simulink model "Vehicle_definitivo_validazione_2"  (R2025b)
settings: Solver=ode4  StartTime=0.0  StopTime=30  FixedStep=0.001  RelTol=1e-3
undefined symbols (not defined in the file): car, new_lotus_bump, new_lotus_roll, new_lotus_steer, posRef, rad, s, Tau_1, Tau_2, Tau_3, Tau_4, yawRef
libraries: aerolibconvert2 x28, simulink_extras x16, simulink x12, slpidlib x2, mpclib x1
(part 3 of 13)

== system Vehicle_definitivo_validazione_2/Con relaxation/Vehicle/Powertrain/Electric Motor ==
  tps_EM : Inport
  omega wheels : Inport  Port=2
  2-D Lookup Table : Lookup_n-D  BreakpointsForDimension1=[0;5415.9399999999996;5455.8699999999999;5494.6300000000001;5524.8000000000002;5801.2200000000003;6194.8599999999997;6620.2799999999997;6996.5;7478.6599999999999;8072.5500000000002;8891.9799999999996;8998.9200000000001;9966.8600000000006;10994.200000000001;11872.6;13016.16;13972.65;15994.85]  BreakpointsForDimension2=[0;0.25;0.29999999999999999;0.34999999999999998;0.40000000000000002;0.45000000000000001;0.5;0.59999999999999998;0.69999999999999996;0.80000000000000004;1]  Table=[0 1.72854705 2.07425646 2.41996587 2.7656752899999999 3.1113846999999999 3.4570941099999999 4.1485129299999999 4.8399317000000002 5.5313505699999999 6.9141880000000002;0 1.72755429 2.0730651500000001 2.4185760100000002 2.7640868599999999 3.10959772 3.4551085800000001 4.1461303000000003 4.8371519999999997 5.5281737299999998 6.9102170000000003;0 1.7172173399999999 2.0606608099999999 2.4041042799999999 2.7475477499999998 3.0909912099999999 3.4344346799999999 4.1213216199999998 4.8082086000000004 5.4950954899999997 6.8688690000000001;0 1.7114327 2.0537192399999999 2.3960057799999999 2.7382923199999998 3.0805788600000001 3.4228654000000001 4.1074384799999999 4.7920116000000004 5.4765846399999996 6.8457309999999998;0 1.7057860899999999 2.0469433100000001 2.3881005200000001 2.72925774 3.0704149599999999 3.4115721799999998 4.0938866100000002 4.7762010000000004 5.45851548 6.8231440000000001;0 1.65353861 1.9842463299999999 2.3149540499999999 2.6456617699999998 2.9763694900000002 3.3070772100000001 3.96849265 4.6299080999999997 5.2913235399999996 6.6141540000000001;0 1.57836584 1.89403901 2.2097121799999999 2.5253853500000001 2.8410585199999998 3.15673168 3.7880780199999999 4.4194243999999996 5.0507707000000002 6.3134629999999996;0 1.5001957400000001 1.80023489 2.10027404 2.4003131899999999 2.7003523399999998 3.0003914800000002 3.6004697800000001 4.2005480999999998 4.8006263699999998 6.0007830000000002;0 1.43080228 1.71696274 2.0031231900000002 2.2892836499999998 2.5754440999999999 2.86160456 3.4339254700000001 4.0062464000000002 4.5785672899999996 5.7232089999999998;0 1.34976662 1.6197199499999999 1.8896732700000001 2.1596266000000002 2.4295799200000001 2.69953325 3.2394398899999999 3.7793464999999999 4.3192531900000004 5.3990660000000004;0 1.24874098 1.49848917 1.74823737 1.99798556 2.24773376 2.4974819500000001 2.9969783400000001 3.4964746999999998 3.9959711200000001 4.9949640000000004;0 1.1245459799999999 1.3494551800000001 1.57436438 1.79927357 2.0241827699999999 2.2490919699999998 2.6989103600000002 3.1487288000000002 3.5985471499999999 4.4981840000000002;0 1.11256427 1.3350771299999999 1.5575899799999999 1.7801028299999999 2.0026156899999998 2.22512854 2.67015425 3.1151800000000001 3.5602056700000002 4.4502569999999997;0 0.98525799000000003 1.18230959 1.3793611800000001 1.5764127800000001 1.7734643800000001 1.9705159800000001 2.3646191700000001 2.7587223999999999 3.1528255600000001 3.9410319999999999;0 0.88127745999999996 1.0575329600000001 1.23378845 1.41004394 1.5862994399999999 1.7625549300000001 2.1150659100000002 2.4675769000000001 2.8200878899999999 3.5251100000000002;0 0.79965012999999996 0.95958014999999997 1.11951018 1.2794402 1.43937023 1.59930025 1.9191602999999999 2.2390203999999998 2.5588804000000001 3.198601;0 0.70417978000000003 0.84501572999999996 0.98585168999999995 1.1266876400000001 1.2675236000000001 1.4083595600000001 1.6900314700000001 1.9717034 2.2533752900000001 2.816719;0 0.63972525999999996 0.76767032000000002 0.89561537000000002 1.0235604199999999 1.15150547 1.2794505300000001 1.5353406300000001 1.7912307000000001 2.0471208399999998 2.5589010000000001;0 0.51010575999999996 0.61212690999999997 0.71414805999999997 0.81616922000000003 0.91819037000000003 1.0202115199999999 1.2242538199999999 1.4282961000000001 1.6323384299999999 2.0404230000000001]  InternalRulePriority=Speed  RndMeth=Simplest
      settings: InputPortMap=u0,u1
  2-D Lookup Table1 : Lookup_n-D  BreakpointsForDimension1=[0;5415.9399999999996;5455.8699999999999;5494.6300000000001;5524.8000000000002;5801.2200000000003;6194.8599999999997;6620.2799999999997;6996.5;7478.6599999999999;8072.5500000000002;8891.9799999999996;8998.9200000000001;9966.8600000000006;10994.200000000001;11872.6;13016.16;13972.65;15994.85]  BreakpointsForDimension2=[0;0.25;0.29999999999999999;0.34999999999999998;0.40000000000000002;0.45000000000000001;0.5;0.59999999999999998;0.69999999999999996;0.80000000000000004;1]  Table=[0 1.72854705 2.07425646 2.41996587 2.7656752899999999 3.1113846999999999 3.4570941099999999 4.1485129299999999 4.8399317000000002 5.5313505699999999 6.9141880000000002;0 1.72755429 2.0730651500000001 2.4185760100000002 2.7640868599999999 3.10959772 3.4551085800000001 4.1461303000000003 4.8371519999999997 5.5281737299999998 6.9102170000000003;0 1.7172173399999999 2.0606608099999999 2.4041042799999999 2.7475477499999998 3.0909912099999999 3.4344346799999999 4.1213216199999998 4.8082086000000004 5.4950954899999997 6.8688690000000001;0 1.7114327 2.0537192399999999 2.3960057799999999 2.7382923199999998 3.0805788600000001 3.4228654000000001 4.1074384799999999 4.7920116000000004 5.4765846399999996 6.8457309999999998;0 1.7057860899999999 2.0469433100000001 2.3881005200000001 2.72925774 3.0704149599999999 3.4115721799999998 4.0938866100000002 4.7762010000000004 5.45851548 6.8231440000000001;0 1.65353861 1.9842463299999999 2.3149540499999999 2.6456617699999998 2.9763694900000002 3.3070772100000001 3.96849265 4.6299080999999997 5.2913235399999996 6.6141540000000001;0 1.57836584 1.89403901 2.2097121799999999 2.5253853500000001 2.8410585199999998 3.15673168 3.7880780199999999 4.4194243999999996 5.0507707000000002 6.3134629999999996;0 1.5001957400000001 1.80023489 2.10027404 2.4003131899999999 2.7003523399999998 3.0003914800000002 3.6004697800000001 4.2005480999999998 4.8006263699999998 6.0007830000000002;0 1.43080228 1.71696274 2.0031231900000002 2.2892836499999998 2.5754440999999999 2.86160456 3.4339254700000001 4.0062464000000002 4.5785672899999996 5.7232089999999998;0 1.34976662 1.6197199499999999 1.8896732700000001 2.1596266000000002 2.4295799200000001 2.69953325 3.2394398899999999 3.7793464999999999 4.3192531900000004 5.3990660000000004;0 1.24874098 1.49848917 1.74823737 1.99798556 2.24773376 2.4974819500000001 2.9969783400000001 3.4964746999999998 3.9959711200000001 4.9949640000000004;0 1.1245459799999999 1.3494551800000001 1.57436438 1.79927357 2.0241827699999999 2.2490919699999998 2.6989103600000002 3.1487288000000002 3.5985471499999999 4.4981840000000002;0 1.11256427 1.3350771299999999 1.5575899799999999 1.7801028299999999 2.0026156899999998 2.22512854 2.67015425 3.1151800000000001 3.5602056700000002 4.4502569999999997;0 0.98525799000000003 1.18230959 1.3793611800000001 1.5764127800000001 1.7734643800000001 1.9705159800000001 2.3646191700000001 2.7587223999999999 3.1528255600000001 3.9410319999999999;0 0.88127745999999996 1.0575329600000001 1.23378845 1.41004394 1.5862994399999999 1.7625549300000001 2.1150659100000002 2.4675769000000001 2.8200878899999999 3.5251100000000002;0 0.79965012999999996 0.95958014999999997 1.11951018 1.2794402 1.43937023 1.59930025 1.9191602999999999 2.2390203999999998 2.5588804000000001 3.198601;0 0.70417978000000003 0.84501572999999996 0.98585168999999995 1.1266876400000001 1.2675236000000001 1.4083595600000001 1.6900314700000001 1.9717034 2.2533752900000001 2.816719;0 0.63972525999999996 0.76767032000000002 0.89561537000000002 1.0235604199999999 1.15150547 1.2794505300000001 1.5353406300000001 1.7912307000000001 2.0471208399999998 2.5589010000000001;0 0.51010575999999996 0.61212690999999997 0.71414805999999997 0.81616922000000003 0.91819037000000003 1.0202115199999999 1.2242538199999999 1.4282961000000001 1.6323384299999999 2.0404230000000001]  InternalRulePriority=Speed  RndMeth=Simplest
      settings: InputPortMap=u0,u1
  Angular Velocity Conversion : aerolibconvert2/Angular Velocity Conversion  IU=rpm  OU=rad/s
  Angular Velocity Conversion1 : aerolibconvert2/Angular Velocity Conversion  IU=rad/s  OU=rpm
  Angular Velocity Conversion2 : aerolibconvert2/Angular Velocity Conversion  IU=rpm  OU=rad/s
  Demux : Demux
  Gain : Gain  Gain=car.Tau_EM
  Gain1 : Gain  Gain=car.Tau_EM
  Gain3 : Gain  Gain=car.Tau_EM
  Integrator : Integrator  InitialCondition=1  LimitOutput=on  UpperSaturationLimit=1  LowerSaturationLimit=0
  Limiter1 : Saturate  UpperLimit=16000  LowerLimit=0
  MATLAB Function : MATLAB Function  TreatAsAtomicUnit=on
  T_FR : Outport
  T_FL : Outport  Port=2
  wires:
  2-D Lookup Table/1 -> Gain/1, MATLAB Function/1(T_FR)
  2-D Lookup Table1/1 -> MATLAB Function/2(T_FL), Gain1/1
  omega wheels/1 -> Angular Velocity Conversion1/1
  Angular Velocity Conversion1/1 -> Gain3/1
  Gain3/1 -> Limiter1/1
  Gain/1 -> T_FR/1
  Gain1/1 -> T_FL/1
  tps_EM/1 -> 2-D Lookup Table1/2, 2-D Lookup Table/2
  Limiter1/1 -> Demux/1
  Demux/1 -> 2-D Lookup Table/1, Angular Velocity Conversion/1
  Demux/2 -> Angular Velocity Conversion2/1, 2-D Lookup Table1/1
  MATLAB Function/1(SoC_dot) -> Integrator/1
  Integrator/1 -> MATLAB Function/5(SoC)
  Angular Velocity Conversion/1 -> MATLAB Function/3(w_FR)
  Angular Velocity Conversion2/1 -> MATLAB Function/4(w_FL)

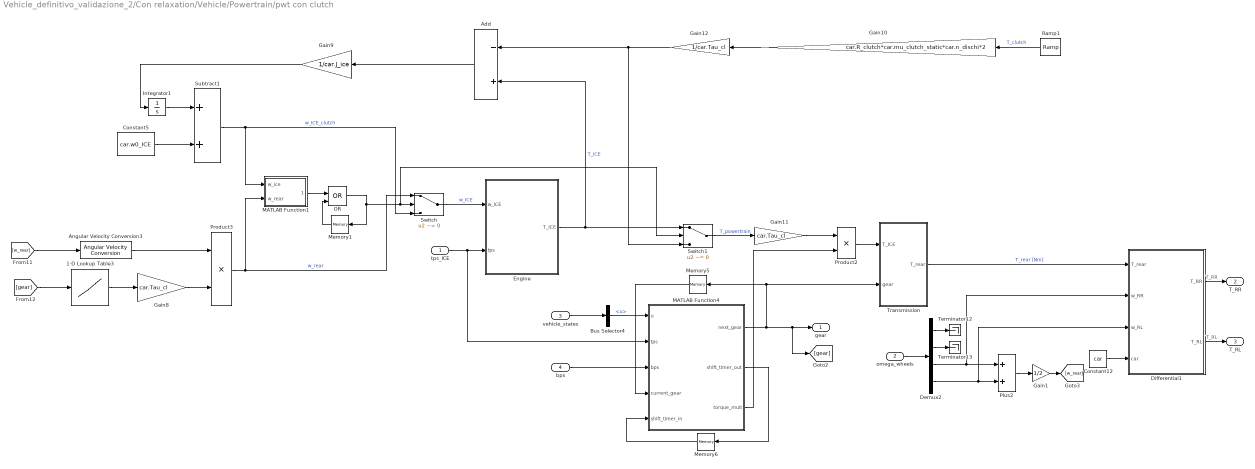
== system Vehicle_definitivo_validazione_2/Con relaxation/Vehicle/Powertrain/pwt con clutch ==
  tps_ICE : Inport
  omega_wheels : Inport  Port=2
  vehicle_states : Inport  Port=3
  bps : Inport  Port=4
  1-D Lookup Table3 : Lookup_n-D  NumberOfTableDimensions=1  BreakpointsForDimension1=[1;2;3;4]  Table=[Tau_1; Tau_2; Tau_3; Tau_4]  InternalRulePriority=Speed  RndMeth=Simplest
  Add : Sum  Inputs=-+
  Angular Velocity Conversion3 : aerolibconvert2/Angular Velocity Conversion  IU=rad/s  OU=rpm
  Bus Selector4 : BusSelector  OutputSignals=velocities.u
  Constant12 : Constant  Value=car  OutDataTypeStr=Bus: slBus1
  Constant5 : Constant  Value=car.w0_ICE
  Demux2 : Demux
  Differential1 : MATLAB Function  TreatAsAtomicUnit=on
  Engine : Subsystem
  Gain1 : Gain  Gain=1/2
  Gain10 : Gain  Gain=car.R_clutch*car.mu_clutch_static*car.n_dischi*2
  Gain11 : Gain  Gain=car.Tau_cl
  Gain12 : Gain  Gain=1/car.Tau_cl
  Gain8 : Gain  Gain=car.Tau_cl
  Gain9 : Gain  Gain=1/car.J_ice
  Integrator1 : Integrator
  MATLAB Function1 : MATLAB Function  TreatAsAtomicUnit=on
  MATLAB Function4 : MATLAB Function  TreatAsAtomicUnit=on
  Memory1 : Memory
  Memory5 : Memory  InitialCondition=2
  Memory6 : Memory
  OR : Logic  Operator=OR  IconShape=distinctive  AllPortsSameDT=off  OutDataTypeStr=boolean
  Plus2 : Sum
  Product2 : Product
  Product3 : Product
  Ramp1 : simulink/Sources/Ramp  slope=5000  start=0  InitialOutput=671
  Subtract1 : Sum
  Switch : Switch  Criteria=u2 ~= 0  Threshold=50  SaturateOnIntegerOverflow=off  InputSameDT=off
  Switch1 : Switch  Criteria=u2 ~= 0  Threshold=50  SaturateOnIntegerOverflow=off  InputSameDT=off
  Terminator12 : Terminator
  Terminator13 : Terminator
  Transmission : Subsystem
  gear : Outport
  T_RR : Outport  Port=2
  T_RL : Outport  Port=3
  wires:
  Ramp1/1 -> Gain10/1  "T_clutch"
  MATLAB Function1/1(condizione) -> OR/1
  [gear] -> 1-D Lookup Table3/1
  Gain10/1 -> Gain12/1
  Angular Velocity Conversion3/1 -> Product3/1
  [w_rear] -> Angular Velocity Conversion3/1
  Gain12/1 -> Switch1/3, Add/1
  Integrator1/1 -> Subtract1/1
  Switch/1 -> Engine/1(w_ICE)  "w_ICE"
  Subtract1/1 -> Switch/3, MATLAB Function1/1(w_ice)  "w_ICE_clutch"
  Switch1/1 -> Gain11/1  "T_powertrain"
  Constant5/1 -> Subtract1/2
  Memory1/1 -> OR/2
  tps_ICE/1 -> Engine/2(tps), MATLAB Function4/2(tps)
  Add/1 -> Gain9/1
  Memory5/1 -> MATLAB Function4/4(current_gear)
  bps/1 -> MATLAB Function4/3(bps)
  OR/1 -> Memory1/1, Switch/2, Switch1/2
  vehicle_states/1 -> Bus Selector4/1
  Demux2/1 -> Terminator12/1
  Gain8/1 -> Product3/2
  Gain1/1 -> [w_rear]
  1-D Lookup Table3/1 -> Gain8/1
  Plus2/1 -> Gain1/1
  omega_wheels/1 -> Demux2/1
  MATLAB Function4/2(shift_timer_out) -> Memory6/1
  Transmission/1(T_rear) -> Differential1/1(T_rear)  "T_rear [Nm]"
  Memory6/1 -> MATLAB Function4/5(shift_timer_in)
  Demux2/2 -> Terminator13/1
  Demux2/4 -> Differential1/3(w_RL), Plus2/2
  Bus Selector4/1 -> MATLAB Function4/1(u)  "<u>"
  Demux2/3 -> Differential1/2(w_RR), Plus2/1
  MATLAB Function4/1(next_gear) -> Memory5/1, Transmission/2(gear), gear/1, [gear]
  Product3/1 -> MATLAB Function1/2(w_rear), Switch/1  "w_rear"
  Gain11/1 -> Product2/1
  MATLAB Function4/3(torque_mult) -> Product2/2
  Engine/1(T_ICE) -> Add/2, Switch1/1  "T_ICE"
  Gain9/1 -> Integrator1/1
  Product2/1 -> Transmission/1(T_ICE)
  Differential1/1(T_RR) -> T_RR/1  "T_RR"
  Constant12/1 -> Differential1/4(car)
  Differential1/2(T_RL) -> T_RL/1  "T_RL"

== system Vehicle_definitivo_validazione_2/Con relaxation/Vehicle/Powertrain/pwt senza clutch ==
  tps_ICE : Inport
  vehicle_states : Inport  Port=2
  bps : Inport  Port=3
  omega_wheels : Inport  Port=4
  1-D Lookup Table1 : Lookup_n-D  NumberOfTableDimensions=1  BreakpointsForDimension1=[1;2;3;4]  Table=[Tau_1; Tau_2; Tau_3; Tau_4]  InternalRulePriority=Speed  RndMeth=Simplest
  Angular Velocity Conversion1 : aerolibconvert2/Angular Velocity Conversion  IU=rad/s  OU=rpm
  Bus Selector3 : BusSelector  OutputSignals=Veh_States.velocities.u
  Constant12 : Constant  Value=car  OutDataTypeStr=Bus: slBus1
  Demux : Demux
  Differential : MATLAB Function  TreatAsAtomicUnit=on
  Engine : Subsystem
  Gain1 : Gain  Gain=1/2
  Gain2 : Gain  Gain=car.Tau_cl
  Gain5 : Gain  Gain=car.Tau_cl
  Gearbox : MATLAB Function  TreatAsAtomicUnit=on
  Memory : Memory  InitialCondition=2
  Memory3 : Memory
  Plus : Sum
  Product : Product
  Product1 : Product
  Terminator : Terminator
  Terminator1 : Terminator
  Transmission : Subsystem
  T_RR : Outport
  T_RL : Outport  Port=2
  gear : Outport  Port=3
  wires:
  Memory/1 -> Gearbox/4(current_gear)
  Gain5/1 -> Product1/2
  vehicle_states/1 -> Bus Selector3/1
  Angular Velocity Conversion1/1 -> Product1/1
  Gearbox/3(shift_timer_out) -> Memory3/1
  Memory3/1 -> Gearbox/5(shift_timer_in)
  bps/1 -> Gearbox/3(bps)  "bps"
  1-D Lookup Table1/1 -> Gain5/1
  Bus Selector3/1 -> Gearbox/1(u)  "<u>"
  Gearbox/1(next_gear) -> Memory/1, Transmission/2(gear), gear/1, [gear]  "gear"
  [gear] -> 1-D Lookup Table1/1
  Transmission/1(T_rear) -> Differential/1(T_rear)  "T_rear [Nm]"
  tps_ICE/1 -> Gearbox/2(tps), Engine/2(tps)  "tps"
  Product/1 -> Transmission/1(T_ICE)
  Engine/1(T_ICE) -> Gain2/1  "T_ICE"
  Product1/1 -> Engine/1(w_ICE)  "w_ICE"
  Gearbox/2(torque_mult) -> Product/2
  Gain2/1 -> Product/1
  Plus/1 -> Gain1/1
  Demux/3 -> Plus/1, [w_RR]
  Gain1/1 -> Angular Velocity Conversion1/1
  Demux/4 -> [w_RL], Plus/2
  omega_wheels/1 -> Demux/1
  Demux/1 -> Terminator/1  "w_front"
  Demux/2 -> Terminator1/1
  Differential/1(T_RR) -> T_RR/1  "T_RR"
  Differential/2(T_RL) -> T_RL/1  "T_RL"
  [w_RR] -> Differential/2(w_RR)
  [w_RL] -> Differential/3(w_RL)
  Constant12/1 -> Differential/4(car)

== system Vehicle_definitivo_validazione_2/Driver in the Loop/Vehicle/Brakes/Front Caliper ==
  P_Front : Inport
  Gain : Gain  Gain=4
  Pad Friction : Gain  Gain=car.brakepad_friction_coeff
  Piston area : Gain  Gain=car.area_front_piston
  brake radius : Gain  Gain=car.brake_radius_front
  from bar to Pascal : Gain  Gain=100000
  T_brake_FR : Outport
  T_brake_FL : Outport  Port=2
  wires:
  P_Front/1 -> from bar to Pascal/1
  Pad Friction/1 -> brake radius/1
  brake radius/1 -> T_brake_FR/1, T_brake_FL/1
  from bar to Pascal/1 -> Gain/1
  Piston area/1 -> Pad Friction/1
  Gain/1 -> Piston area/1

== system Vehicle_definitivo_validazione_2/Driver in the Loop/Vehicle/Brakes/Proportional Valve ==
  P_rear : Inport
  2-D Lookup Table : Lookup_n-D  BreakpointsForDimension1=[0;3.4473799999999999;6.8947599999999998;10.342140000000001;13.78952;17.236899999999999;20.684280000000001;24.13166;27.579039999999999;31.026420000000002;34.473799999999997;37.92118;41.368560000000002;44.815939999999998;48.26332;51.710700000000003;55.158079999999998;58.605460000000001;62.052840000000003;65.500219999999999;68.947599999999994;72.394980000000004;75.842359999999999;79.289739999999995;82.737120000000004]  BreakpointsForDimension2=[1;2;3;4;5;6;7]  Table=[0 0 0 0 0 0 0;3.4473799999999999 3.4473799999999999 3.4473799999999999 3.4473799999999999 3.4473799999999999 3.4473799999999999 3.4473799999999999;6.8947599999999998 6.8947599999999998 6.8947599999999998 6.8947599999999998 6.8947599999999998 6.8947599999999998 6.8947599999999998;10.342140000000001 10.342140000000001 10.342140000000001 10.342140000000001 10.342140000000001 10.342140000000001 10.342140000000001;11.49126667 13.78952 13.78952 13.78952 13.78952 13.78952 13.78952;12.64039333 17.236899999999999 17.236899999999999 17.236899999999999 17.236899999999999 17.236899999999999 17.236899999999999;13.78952 20.684280000000001 20.684280000000001 20.684280000000001 20.684280000000001 20.684280000000001 20.684280000000001;14.938646670000001 21.833406669999999 24.13166 24.13166 24.13166 24.13166 24.13166;16.087773330000001 22.982533329999999 27.579039999999999 27.579039999999999 27.579039999999999 27.579039999999999 27.579039999999999;17.236899999999999 24.13166 31.026420000000002 31.026420000000002 31.026420000000002 31.026420000000002 31.026420000000002;18.38602667 25.280786670000001 34.473799999999997 34.473799999999997 34.473799999999997 34.473799999999997 34.473799999999997;19.53515333 26.429913330000002 35.458765710000002 37.92118 37.92118 37.92118 37.92118;20.684280000000001 27.579039999999999 36.44373143 41.368560000000002 41.368560000000002 41.368560000000002 41.368560000000002;21.833406669999999 28.72816667 37.428697139999997 42.517686670000003 44.815939999999998 44.815939999999998 44.815939999999998;22.982533329999999 29.877293330000001 38.413662860000002 43.666813329999997 48.26332 48.26332 48.26332;24.13166 31.026420000000002 39.39862857 44.815939999999998 51.710700000000003 51.710700000000003 51.710700000000003;25.280786670000001 32.175546670000003 40.383594289999998 45.965066669999999 52.859826669999997 55.158079999999998 55.158079999999998;26.429913330000002 33.324673330000003 41.368560000000002 47.114193329999999 54.008953329999997 58.605460000000001 58.605460000000001;27.579039999999999 34.473799999999997 42.35352571 48.26332 55.158079999999998 62.052840000000003 62.052840000000003;28.72816667 35.622926669999998 43.338491429999998 49.412446670000001 56.307206669999999 63.201966669999997 65.500219999999999;29.877293330000001 36.772053329999999 44.323457140000002 50.561573330000002 57.45633333 64.351093329999998 68.947599999999994;31.026420000000002 37.92118 45.30842286 51.710700000000003 58.605460000000001 65.500219999999999 70.671289999999999;32.175546670000003 39.070306670000001 46.293388569999998 52.859826669999997 59.754586670000002 66.64934667 72.394980000000004;33.324673330000003 40.219433330000001 47.278354290000003 54.008953329999997 60.903713330000002 67.798473329999993 74.118669999999995;34.473799999999997 41.368560000000002 48.26332 55.158079999999998 62.052840000000003 68.947599999999994 75.842359999999999]  InternalRulePriority=Speed  RndMeth=Simplest
      settings: InputPortMap=u0,u1
  Constant : Constant  Value=car.prop_valve_pos
  p_rear_mod : Outport
  wires:
  P_rear/1 -> 2-D Lookup Table/1
  Constant/1 -> 2-D Lookup Table/2
  2-D Lookup Table/1 -> p_rear_mod/1

== system Vehicle_definitivo_validazione_2/Driver in the Loop/Vehicle/Brakes/Rear Caliper ==
  P_rear : Inport
  Gain : Gain  Gain=2
  Pad Friction : Gain  Gain=car.brakepad_friction_coeff
  Piston area : Gain  Gain=car.area_rear_piston
  brake radius_rear : Gain  Gain=car.brake_radius_rear
  from bar to Pascal : Gain  Gain=100000
  T_brake_RR : Outport
  T_brake_RL : Outport  Port=2
  wires:
  P_rear/1 -> from bar to Pascal/1
  Pad Friction/1 -> brake radius_rear/1
  brake radius_rear/1 -> T_brake_RL/1, T_brake_RR/1
  from bar to Pascal/1 -> Gain/1
  Gain/1 -> Piston area/1
  Piston area/1 -> Pad Friction/1

== system Vehicle_definitivo_validazione_2/Driver in the Loop/Vehicle/Chassis/Aeromaps ==
  Ride_height : Inport
  Constant : Constant  Value=car.Cx
  Constant1 : Constant  Value=car.Cz
  Constant2 : Constant  Value=car.x_cp
  Demux : Demux
  Mux : Mux  Inputs=3
  aero_coeff : Outport
  wires:
  Constant/1 -> Mux/1
  Constant1/1 -> Mux/2
  Ride_height/1 -> Demux/1
  Mux/1 -> aero_coeff/1
  Constant2/1 -> Mux/3

== system Vehicle_definitivo_validazione_2/Driver in the Loop/Vehicle/Chassis/Damper ==
  susp_vel_ground : Inport
  IR : Inport  Port=2
  Demux : Demux
  FL : Subsystem
  FR : Subsystem
  Mux : Mux
  Product : Product
  Product1 : Product
  RL : Subsystem
  RR : Subsystem
  F_damper : Outport
  wires:
  IR/1 -> Product1/2, Product/2
  Product/1 -> Demux/1
  Demux/1 -> FR/1(V_FR)
  FR/1(F_FR) -> Mux/1  "F_FR"
  Mux/1 -> Product1/1
  Demux/2 -> FL/1(V_FL)
  FL/1(F_FL) -> Mux/2  "F_FL"
  Demux/3 -> RR/1(V_RR)
  RR/1(F_RR) -> Mux/3  "F_RR"
  Demux/4 -> RL/1(V_RL)
  RL/1(F_RL) -> Mux/4  "F_RL"
  susp_vel_ground/1 -> Product/1
  Product1/1 -> F_damper/1

== system Vehicle_definitivo_validazione_2/Driver in the Loop/Vehicle/Chassis/kinematics ==
  Steer_Angle : Inport
  Wheel_Travel : Inport  Port=2
  Add{,1..5} (6 alike) : Sum
  Constant : Constant  Value=car.lf
  Constant1 : Constant  Value=car.lr
  Constant2 : Constant  Value=car.h_cog
  Constant3 : Constant  Value=0.03
  Constant4 : Constant  Value=0.04
  Degrees to Radians : simulink_extras/Transformations/Degrees to Radians
  Demux : Demux
  FL : Subsystem
  FR : Subsystem
  Gain{,1..3} (4 alike) : Gain  Gain=0.5
  Gain4 : Gain  Gain=-1
  Mux : Mux  Inputs=11
  Mux1 : Mux
  Mux2 : Mux
  Mux3 : Mux
  RL : Subsystem
  RR : Subsystem
  Subsystem : Subsystem
  Subsystem1 : Subsystem
  Subtract : Sum  Inputs=-+
  Subtract1 : Sum  Inputs=-+
  kin_dyn : Outport
  anti% : Outport  Port=2
  camber : Outport  Port=3
  toe : Outport  Port=4
  wires:
  Demux/1 -> FR/1(Wheel_Travel), Subtract/1, Add/1
  Add/1 -> Gain/1
  Gain/1 -> Subsystem/1(Heave_F)
  Subtract/1 -> Subsystem/2(Roll_F)
  Demux/3 -> Subtract1/1, Add1/1, RR/1(Wheel_Travel)
  Demux/4 -> RL/1(Wheel_Travel), Add1/2, Subtract1/2
  Add1/1 -> Gain1/1
  Steer_Angle/1 -> FR/2(Steer_Angle), Gain4/1
  Demux/2 -> FL/2(Wheel_Travel), Add/2, Subtract/2
  Mux/1 -> kin_dyn/1
  FR/3(IR_FR) -> Mux/1
  FL/3(IR_FL) -> Mux/2
  RR/3(IR_RR) -> Mux/3
  RL/3(IR_RL) -> Mux/4
  Subsystem/2(tf) -> Mux/5
  Subsystem1/2(tr) -> Mux/6
  FR/1(wb_FR) -> Add2/1
  FL/1(wb_FL) -> Add2/2
  Add2/1 -> Gain2/1
  Gain2/1 -> Add3/1
  Constant/1 -> Add3/2
  Add3/1 -> Mux/7
  Constant1/1 -> Add5/2
  Gain3/1 -> Add5/1
  Add4/1 -> Gain3/1
  Add5/1 -> Mux/8
  RR/1(wb_RR) -> Add4/1
  RL/1(wb_RL) -> Add4/2
  Constant2/1 -> Mux/9
  Mux3/1 -> Degrees to Radians/1
  Mux2/1 -> camber/1
  Mux1/1 -> anti%/1
  FR/2(AD_FR) -> Mux1/1
  FL/2(AD_FL) -> Mux1/2
  RR/2(AS_RR) -> Mux1/3
  RL/2(AS_RL) -> Mux1/4
  FR/4(Camber_FR) -> Mux2/1
  FL/4(Camber_FL) -> Mux2/2
  RR/4(Camber_RR) -> Mux2/3
  RL/4(Camber_RL) -> Mux2/4
  FR/5(Toe_FR) -> Mux3/1
  FL/5(Toe_FL) -> Mux3/2
  RR/5(Toe_RR) -> Mux3/3
  RL/5(Toe_RL) -> Mux3/4
  Gain4/1 -> FL/1(Steer_Angle)
  Constant3/1 -> Mux/10
  Constant4/1 -> Mux/11
  Subtract1/1 -> Subsystem1/2(Roll_R)
  Gain1/1 -> Subsystem1/1(Heave_R)
  Degrees to Radians/1 -> toe/1
  Wheel_Travel/1 -> Demux/1

== system Vehicle_definitivo_validazione_2/Driver in the Loop/Vehicle/Powertrain/Electric Motor ==
  tps_EM : Inport
  omega wheels : Inport  Port=2
  2-D Lookup Table : Lookup_n-D  BreakpointsForDimension1=[0;5415.9399999999996;5455.8699999999999;5494.6300000000001;5524.8000000000002;5801.2200000000003;6194.8599999999997;6620.2799999999997;6996.5;7478.6599999999999;8072.5500000000002;8891.9799999999996;8998.9200000000001;9966.8600000000006;10994.200000000001;11872.6;13016.16;13972.65;15994.85]  BreakpointsForDimension2=[0;0.25;0.29999999999999999;0.34999999999999998;0.40000000000000002;0.45000000000000001;0.5;0.59999999999999998;0.69999999999999996;0.80000000000000004;1]  Table=[0 1.72854705 2.07425646 2.41996587 2.7656752899999999 3.1113846999999999 3.4570941099999999 4.1485129299999999 4.8399317000000002 5.5313505699999999 6.9141880000000002;0 1.72755429 2.0730651500000001 2.4185760100000002 2.7640868599999999 3.10959772 3.4551085800000001 4.1461303000000003 4.8371519999999997 5.5281737299999998 6.9102170000000003;0 1.7172173399999999 2.0606608099999999 2.4041042799999999 2.7475477499999998 3.0909912099999999 3.4344346799999999 4.1213216199999998 4.8082086000000004 5.4950954899999997 6.8688690000000001;0 1.7114327 2.0537192399999999 2.3960057799999999 2.7382923199999998 3.0805788600000001 3.4228654000000001 4.1074384799999999 4.7920116000000004 5.4765846399999996 6.8457309999999998;0 1.7057860899999999 2.0469433100000001 2.3881005200000001 2.72925774 3.0704149599999999 3.4115721799999998 4.0938866100000002 4.7762010000000004 5.45851548 6.8231440000000001;0 1.65353861 1.9842463299999999 2.3149540499999999 2.6456617699999998 2.9763694900000002 3.3070772100000001 3.96849265 4.6299080999999997 5.2913235399999996 6.6141540000000001;0 1.57836584 1.89403901 2.2097121799999999 2.5253853500000001 2.8410585199999998 3.15673168 3.7880780199999999 4.4194243999999996 5.0507707000000002 6.3134629999999996;0 1.5001957400000001 1.80023489 2.10027404 2.4003131899999999 2.7003523399999998 3.0003914800000002 3.6004697800000001 4.2005480999999998 4.8006263699999998 6.0007830000000002;0 1.43080228 1.71696274 2.0031231900000002 2.2892836499999998 2.5754440999999999 2.86160456 3.4339254700000001 4.0062464000000002 4.5785672899999996 5.7232089999999998;0 1.34976662 1.6197199499999999 1.8896732700000001 2.1596266000000002 2.4295799200000001 2.69953325 3.2394398899999999 3.7793464999999999 4.3192531900000004 5.3990660000000004;0 1.24874098 1.49848917 1.74823737 1.99798556 2.24773376 2.4974819500000001 2.9969783400000001 3.4964746999999998 3.9959711200000001 4.9949640000000004;0 1.1245459799999999 1.3494551800000001 1.57436438 1.79927357 2.0241827699999999 2.2490919699999998 2.6989103600000002 3.1487288000000002 3.5985471499999999 4.4981840000000002;0 1.11256427 1.3350771299999999 1.5575899799999999 1.7801028299999999 2.0026156899999998 2.22512854 2.67015425 3.1151800000000001 3.5602056700000002 4.4502569999999997;0 0.98525799000000003 1.18230959 1.3793611800000001 1.5764127800000001 1.7734643800000001 1.9705159800000001 2.3646191700000001 2.7587223999999999 3.1528255600000001 3.9410319999999999;0 0.88127745999999996 1.0575329600000001 1.23378845 1.41004394 1.5862994399999999 1.7625549300000001 2.1150659100000002 2.4675769000000001 2.8200878899999999 3.5251100000000002;0 0.79965012999999996 0.95958014999999997 1.11951018 1.2794402 1.43937023 1.59930025 1.9191602999999999 2.2390203999999998 2.5588804000000001 3.198601;0 0.70417978000000003 0.84501572999999996 0.98585168999999995 1.1266876400000001 1.2675236000000001 1.4083595600000001 1.6900314700000001 1.9717034 2.2533752900000001 2.816719;0 0.63972525999999996 0.76767032000000002 0.89561537000000002 1.0235604199999999 1.15150547 1.2794505300000001 1.5353406300000001 1.7912307000000001 2.0471208399999998 2.5589010000000001;0 0.51010575999999996 0.61212690999999997 0.71414805999999997 0.81616922000000003 0.91819037000000003 1.0202115199999999 1.2242538199999999 1.4282961000000001 1.6323384299999999 2.0404230000000001]  InternalRulePriority=Speed  RndMeth=Simplest
      settings: InputPortMap=u0,u1
  2-D Lookup Table1 : Lookup_n-D  BreakpointsForDimension1=[0;5415.9399999999996;5455.8699999999999;5494.6300000000001;5524.8000000000002;5801.2200000000003;6194.8599999999997;6620.2799999999997;6996.5;7478.6599999999999;8072.5500000000002;8891.9799999999996;8998.9200000000001;9966.8600000000006;10994.200000000001;11872.6;13016.16;13972.65;15994.85]  BreakpointsForDimension2=[0;0.25;0.29999999999999999;0.34999999999999998;0.40000000000000002;0.45000000000000001;0.5;0.59999999999999998;0.69999999999999996;0.80000000000000004;1]  Table=[0 1.72854705 2.07425646 2.41996587 2.7656752899999999 3.1113846999999999 3.4570941099999999 4.1485129299999999 4.8399317000000002 5.5313505699999999 6.9141880000000002;0 1.72755429 2.0730651500000001 2.4185760100000002 2.7640868599999999 3.10959772 3.4551085800000001 4.1461303000000003 4.8371519999999997 5.5281737299999998 6.9102170000000003;0 1.7172173399999999 2.0606608099999999 2.4041042799999999 2.7475477499999998 3.0909912099999999 3.4344346799999999 4.1213216199999998 4.8082086000000004 5.4950954899999997 6.8688690000000001;0 1.7114327 2.0537192399999999 2.3960057799999999 2.7382923199999998 3.0805788600000001 3.4228654000000001 4.1074384799999999 4.7920116000000004 5.4765846399999996 6.8457309999999998;0 1.7057860899999999 2.0469433100000001 2.3881005200000001 2.72925774 3.0704149599999999 3.4115721799999998 4.0938866100000002 4.7762010000000004 5.45851548 6.8231440000000001;0 1.65353861 1.9842463299999999 2.3149540499999999 2.6456617699999998 2.9763694900000002 3.3070772100000001 3.96849265 4.6299080999999997 5.2913235399999996 6.6141540000000001;0 1.57836584 1.89403901 2.2097121799999999 2.5253853500000001 2.8410585199999998 3.15673168 3.7880780199999999 4.4194243999999996 5.0507707000000002 6.3134629999999996;0 1.5001957400000001 1.80023489 2.10027404 2.4003131899999999 2.7003523399999998 3.0003914800000002 3.6004697800000001 4.2005480999999998 4.8006263699999998 6.0007830000000002;0 1.43080228 1.71696274 2.0031231900000002 2.2892836499999998 2.5754440999999999 2.86160456 3.4339254700000001 4.0062464000000002 4.5785672899999996 5.7232089999999998;0 1.34976662 1.6197199499999999 1.8896732700000001 2.1596266000000002 2.4295799200000001 2.69953325 3.2394398899999999 3.7793464999999999 4.3192531900000004 5.3990660000000004;0 1.24874098 1.49848917 1.74823737 1.99798556 2.24773376 2.4974819500000001 2.9969783400000001 3.4964746999999998 3.9959711200000001 4.9949640000000004;0 1.1245459799999999 1.3494551800000001 1.57436438 1.79927357 2.0241827699999999 2.2490919699999998 2.6989103600000002 3.1487288000000002 3.5985471499999999 4.4981840000000002;0 1.11256427 1.3350771299999999 1.5575899799999999 1.7801028299999999 2.0026156899999998 2.22512854 2.67015425 3.1151800000000001 3.5602056700000002 4.4502569999999997;0 0.98525799000000003 1.18230959 1.3793611800000001 1.5764127800000001 1.7734643800000001 1.9705159800000001 2.3646191700000001 2.7587223999999999 3.1528255600000001 3.9410319999999999;0 0.88127745999999996 1.0575329600000001 1.23378845 1.41004394 1.5862994399999999 1.7625549300000001 2.1150659100000002 2.4675769000000001 2.8200878899999999 3.5251100000000002;0 0.79965012999999996 0.95958014999999997 1.11951018 1.2794402 1.43937023 1.59930025 1.9191602999999999 2.2390203999999998 2.5588804000000001 3.198601;0 0.70417978000000003 0.84501572999999996 0.98585168999999995 1.1266876400000001 1.2675236000000001 1.4083595600000001 1.6900314700000001 1.9717034 2.2533752900000001 2.816719;0 0.63972525999999996 0.76767032000000002 0.89561537000000002 1.0235604199999999 1.15150547 1.2794505300000001 1.5353406300000001 1.7912307000000001 2.0471208399999998 2.5589010000000001;0 0.51010575999999996 0.61212690999999997 0.71414805999999997 0.81616922000000003 0.91819037000000003 1.0202115199999999 1.2242538199999999 1.4282961000000001 1.6323384299999999 2.0404230000000001]  InternalRulePriority=Speed  RndMeth=Simplest
      settings: InputPortMap=u0,u1
  Angular Velocity Conversion : aerolibconvert2/Angular Velocity Conversion  IU=rpm  OU=rad/s
  Angular Velocity Conversion1 : aerolibconvert2/Angular Velocity Conversion  IU=rad/s  OU=rpm
  Angular Velocity Conversion2 : aerolibconvert2/Angular Velocity Conversion  IU=rpm  OU=rad/s
  Demux : Demux
  Gain : Gain  Gain=car.Tau_EM
  Gain1 : Gain  Gain=car.Tau_EM
  Gain3 : Gain  Gain=car.Tau_EM
  Integrator : Integrator  InitialCondition=1  LimitOutput=on  UpperSaturationLimit=1  LowerSaturationLimit=0
  Limiter1 : Saturate  UpperLimit=16000  LowerLimit=0
  MATLAB Function : MATLAB Function  TreatAsAtomicUnit=on
  T_FR : Outport
  T_FL : Outport  Port=2
  wires:
  2-D Lookup Table/1 -> Gain/1, MATLAB Function/1(T_FR)
  2-D Lookup Table1/1 -> MATLAB Function/2(T_FL), Gain1/1
  omega wheels/1 -> Angular Velocity Conversion1/1
  Angular Velocity Conversion1/1 -> Gain3/1
  Gain3/1 -> Limiter1/1
  Gain/1 -> T_FR/1
  Gain1/1 -> T_FL/1
  tps_EM/1 -> 2-D Lookup Table1/2, 2-D Lookup Table/2
  Limiter1/1 -> Demux/1
  Demux/1 -> 2-D Lookup Table/1, Angular Velocity Conversion/1
  Demux/2 -> Angular Velocity Conversion2/1, 2-D Lookup Table1/1
  MATLAB Function/1(SoC_dot) -> Integrator/1
  Integrator/1 -> MATLAB Function/5(SoC)
  Angular Velocity Conversion/1 -> MATLAB Function/3(w_FR)
  Angular Velocity Conversion2/1 -> MATLAB Function/4(w_FL)

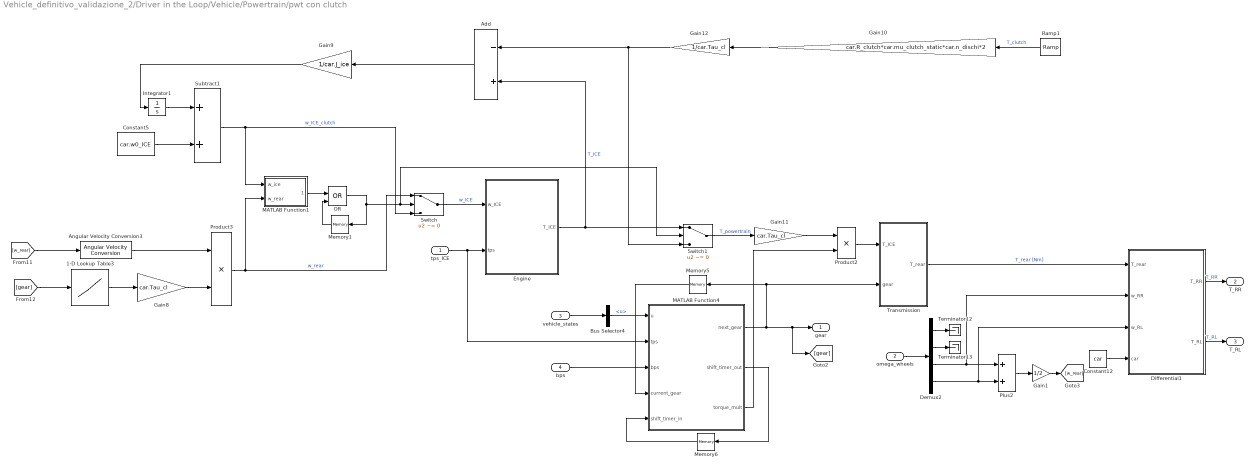
== system Vehicle_definitivo_validazione_2/Driver in the Loop/Vehicle/Powertrain/pwt con clutch ==
  tps_ICE : Inport
  omega_wheels : Inport  Port=2
  vehicle_states : Inport  Port=3
  bps : Inport  Port=4
  1-D Lookup Table3 : Lookup_n-D  NumberOfTableDimensions=1  BreakpointsForDimension1=[1;2;3;4]  Table=[Tau_1; Tau_2; Tau_3; Tau_4]  InternalRulePriority=Speed  RndMeth=Simplest
  Add : Sum  Inputs=-+
  Angular Velocity Conversion3 : aerolibconvert2/Angular Velocity Conversion  IU=rad/s  OU=rpm
  Bus Selector4 : BusSelector  OutputSignals=velocities.u
  Constant12 : Constant  Value=car  OutDataTypeStr=Bus: slBus1
  Constant5 : Constant  Value=car.w0_ICE
  Demux2 : Demux
  Differential1 : MATLAB Function  TreatAsAtomicUnit=on
  Engine : Subsystem
  Gain1 : Gain  Gain=1/2
  Gain10 : Gain  Gain=car.R_clutch*car.mu_clutch_static*car.n_dischi*2
  Gain11 : Gain  Gain=car.Tau_cl
  Gain12 : Gain  Gain=1/car.Tau_cl
  Gain8 : Gain  Gain=car.Tau_cl
  Gain9 : Gain  Gain=1/car.J_ice
  Integrator1 : Integrator
  MATLAB Function1 : MATLAB Function  TreatAsAtomicUnit=on
  MATLAB Function4 : MATLAB Function  TreatAsAtomicUnit=on
  Memory1 : Memory
  Memory5 : Memory  InitialCondition=2
  Memory6 : Memory
  OR : Logic  Operator=OR  IconShape=distinctive  AllPortsSameDT=off  OutDataTypeStr=boolean
  Plus2 : Sum
  Product2 : Product
  Product3 : Product
  Ramp1 : simulink/Sources/Ramp  slope=5000  start=0  InitialOutput=671
  Subtract1 : Sum
  Switch : Switch  Criteria=u2 ~= 0  Threshold=50  SaturateOnIntegerOverflow=off  InputSameDT=off
  Switch1 : Switch  Criteria=u2 ~= 0  Threshold=50  SaturateOnIntegerOverflow=off  InputSameDT=off
  Terminator12 : Terminator
  Terminator13 : Terminator
  Transmission : Subsystem
  gear : Outport
  T_RR : Outport  Port=2
  T_RL : Outport  Port=3
  wires:
  Ramp1/1 -> Gain10/1  "T_clutch"
  MATLAB Function1/1(condizione) -> OR/1
  [gear] -> 1-D Lookup Table3/1
  Gain10/1 -> Gain12/1
  Angular Velocity Conversion3/1 -> Product3/1
  [w_rear] -> Angular Velocity Conversion3/1
  Gain12/1 -> Switch1/3, Add/1
  Integrator1/1 -> Subtract1/1
  Switch/1 -> Engine/1(w_ICE)  "w_ICE"
  Subtract1/1 -> Switch/3, MATLAB Function1/1(w_ice)  "w_ICE_clutch"
  Switch1/1 -> Gain11/1  "T_powertrain"
  Constant5/1 -> Subtract1/2
  Memory1/1 -> OR/2
  tps_ICE/1 -> Engine/2(tps), MATLAB Function4/2(tps)
  Add/1 -> Gain9/1
  Memory5/1 -> MATLAB Function4/4(current_gear)
  bps/1 -> MATLAB Function4/3(bps)
  OR/1 -> Memory1/1, Switch/2, Switch1/2
  vehicle_states/1 -> Bus Selector4/1
  Demux2/1 -> Terminator12/1
  Gain8/1 -> Product3/2
  Gain1/1 -> [w_rear]
  1-D Lookup Table3/1 -> Gain8/1
  Plus2/1 -> Gain1/1
  omega_wheels/1 -> Demux2/1
  MATLAB Function4/2(shift_timer_out) -> Memory6/1
  Transmission/1(T_rear) -> Differential1/1(T_rear)  "T_rear [Nm]"
  Memory6/1 -> MATLAB Function4/5(shift_timer_in)
  Demux2/2 -> Terminator13/1
  Demux2/4 -> Differential1/3(w_RL), Plus2/2
  Bus Selector4/1 -> MATLAB Function4/1(u)  "<u>"
  Demux2/3 -> Differential1/2(w_RR), Plus2/1
  MATLAB Function4/1(next_gear) -> Memory5/1, Transmission/2(gear), gear/1, [gear]
  Product3/1 -> MATLAB Function1/2(w_rear), Switch/1  "w_rear"
  Gain11/1 -> Product2/1
  MATLAB Function4/3(torque_mult) -> Product2/2
  Engine/1(T_ICE) -> Add/2, Switch1/1  "T_ICE"
  Gain9/1 -> Integrator1/1
  Product2/1 -> Transmission/1(T_ICE)
  Differential1/1(T_RR) -> T_RR/1  "T_RR"
  Constant12/1 -> Differential1/4(car)
  Differential1/2(T_RL) -> T_RL/1  "T_RL"

== system Vehicle_definitivo_validazione_2/Driver in the Loop/Vehicle/Powertrain/pwt senza clutch ==
  tps_ICE : Inport
  vehicle_states : Inport  Port=2
  bps : Inport  Port=3
  omega_wheels : Inport  Port=4
  1-D Lookup Table1 : Lookup_n-D  NumberOfTableDimensions=1  BreakpointsForDimension1=[1;2;3;4]  Table=[Tau_1; Tau_2; Tau_3; Tau_4]  InternalRulePriority=Speed  RndMeth=Simplest
  Angular Velocity Conversion1 : aerolibconvert2/Angular Velocity Conversion  IU=rad/s  OU=rpm
  Bus Selector3 : BusSelector  OutputSignals=Veh_States.velocities.u
  Constant12 : Constant  Value=car  OutDataTypeStr=Bus: slBus1
  Demux : Demux
  Differential : MATLAB Function  TreatAsAtomicUnit=on
  Engine : Subsystem
  Gain1 : Gain  Gain=1/2
  Gain2 : Gain  Gain=car.Tau_cl
  Gain5 : Gain  Gain=car.Tau_cl
  Gearbox : MATLAB Function  TreatAsAtomicUnit=on
  Memory : Memory  InitialCondition=2
  Memory3 : Memory
  Plus : Sum
  Product : Product
  Product1 : Product
  Terminator : Terminator
  Terminator1 : Terminator
  Transmission : Subsystem
  T_RR : Outport
  T_RL : Outport  Port=2
  gear : Outport  Port=3
  wires:
  Memory/1 -> Gearbox/4(current_gear)
  Gain5/1 -> Product1/2
  vehicle_states/1 -> Bus Selector3/1
  Angular Velocity Conversion1/1 -> Product1/1
  Gearbox/3(shift_timer_out) -> Memory3/1
  Memory3/1 -> Gearbox/5(shift_timer_in)
  bps/1 -> Gearbox/3(bps)  "bps"
  1-D Lookup Table1/1 -> Gain5/1
  Bus Selector3/1 -> Gearbox/1(u)  "<u>"
  Gearbox/1(next_gear) -> Memory/1, Transmission/2(gear), gear/1, [gear]  "gear"
  [gear] -> 1-D Lookup Table1/1
  Transmission/1(T_rear) -> Differential/1(T_rear)  "T_rear [Nm]"
  tps_ICE/1 -> Gearbox/2(tps), Engine/2(tps)  "tps"
  Product/1 -> Transmission/1(T_ICE)
  Engine/1(T_ICE) -> Gain2/1  "T_ICE"
  Product1/1 -> Engine/1(w_ICE)  "w_ICE"
  Gearbox/2(torque_mult) -> Product/2
  Gain2/1 -> Product/1
  Plus/1 -> Gain1/1
  Demux/3 -> Plus/1, [w_RR]
  Gain1/1 -> Angular Velocity Conversion1/1
  Demux/4 -> [w_RL], Plus/2
  omega_wheels/1 -> Demux/1
  Demux/1 -> Terminator/1  "w_front"
  Demux/2 -> Terminator1/1
  Differential/1(T_RR) -> T_RR/1  "T_RR"
  Differential/2(T_RL) -> T_RL/1  "T_RL"
  [w_RR] -> Differential/2(w_RR)
  [w_RL] -> Differential/3(w_RL)
  Constant12/1 -> Differential/4(car)

== system Vehicle_definitivo_validazione_2/Hardware in the Loop/Vehicle/Brakes/Front Caliper ==
  P_Front : Inport
  Gain : Gain  Gain=4
  Pad Friction : Gain  Gain=car.brakepad_friction_coeff
  Piston area : Gain  Gain=car.area_front_piston
  brake radius : Gain  Gain=car.brake_radius_front
  from bar to Pascal : Gain  Gain=100000
  T_brake_FR : Outport
  T_brake_FL : Outport  Port=2
  wires:
  P_Front/1 -> from bar to Pascal/1
  Pad Friction/1 -> brake radius/1
  brake radius/1 -> T_brake_FR/1, T_brake_FL/1
  from bar to Pascal/1 -> Gain/1
  Piston area/1 -> Pad Friction/1
  Gain/1 -> Piston area/1

== system Vehicle_definitivo_validazione_2/Hardware in the Loop/Vehicle/Brakes/Proportional Valve ==
  P_rear : Inport
  2-D Lookup Table : Lookup_n-D  BreakpointsForDimension1=[0;3.4473799999999999;6.8947599999999998;10.342140000000001;13.78952;17.236899999999999;20.684280000000001;24.13166;27.579039999999999;31.026420000000002;34.473799999999997;37.92118;41.368560000000002;44.815939999999998;48.26332;51.710700000000003;55.158079999999998;58.605460000000001;62.052840000000003;65.500219999999999;68.947599999999994;72.394980000000004;75.842359999999999;79.289739999999995;82.737120000000004]  BreakpointsForDimension2=[1;2;3;4;5;6;7]  Table=[0 0 0 0 0 0 0;3.4473799999999999 3.4473799999999999 3.4473799999999999 3.4473799999999999 3.4473799999999999 3.4473799999999999 3.4473799999999999;6.8947599999999998 6.8947599999999998 6.8947599999999998 6.8947599999999998 6.8947599999999998 6.8947599999999998 6.8947599999999998;10.342140000000001 10.342140000000001 10.342140000000001 10.342140000000001 10.342140000000001 10.342140000000001 10.342140000000001;11.49126667 13.78952 13.78952 13.78952 13.78952 13.78952 13.78952;12.64039333 17.236899999999999 17.236899999999999 17.236899999999999 17.236899999999999 17.236899999999999 17.236899999999999;13.78952 20.684280000000001 20.684280000000001 20.684280000000001 20.684280000000001 20.684280000000001 20.684280000000001;14.938646670000001 21.833406669999999 24.13166 24.13166 24.13166 24.13166 24.13166;16.087773330000001 22.982533329999999 27.579039999999999 27.579039999999999 27.579039999999999 27.579039999999999 27.579039999999999;17.236899999999999 24.13166 31.026420000000002 31.026420000000002 31.026420000000002 31.026420000000002 31.026420000000002;18.38602667 25.280786670000001 34.473799999999997 34.473799999999997 34.473799999999997 34.473799999999997 34.473799999999997;19.53515333 26.429913330000002 35.458765710000002 37.92118 37.92118 37.92118 37.92118;20.684280000000001 27.579039999999999 36.44373143 41.368560000000002 41.368560000000002 41.368560000000002 41.368560000000002;21.833406669999999 28.72816667 37.428697139999997 42.517686670000003 44.815939999999998 44.815939999999998 44.815939999999998;22.982533329999999 29.877293330000001 38.413662860000002 43.666813329999997 48.26332 48.26332 48.26332;24.13166 31.026420000000002 39.39862857 44.815939999999998 51.710700000000003 51.710700000000003 51.710700000000003;25.280786670000001 32.175546670000003 40.383594289999998 45.965066669999999 52.859826669999997 55.158079999999998 55.158079999999998;26.429913330000002 33.324673330000003 41.368560000000002 47.114193329999999 54.008953329999997 58.605460000000001 58.605460000000001;27.579039999999999 34.473799999999997 42.35352571 48.26332 55.158079999999998 62.052840000000003 62.052840000000003;28.72816667 35.622926669999998 43.338491429999998 49.412446670000001 56.307206669999999 63.201966669999997 65.500219999999999;29.877293330000001 36.772053329999999 44.323457140000002 50.561573330000002 57.45633333 64.351093329999998 68.947599999999994;31.026420000000002 37.92118 45.30842286 51.710700000000003 58.605460000000001 65.500219999999999 70.671289999999999;32.175546670000003 39.070306670000001 46.293388569999998 52.859826669999997 59.754586670000002 66.64934667 72.394980000000004;33.324673330000003 40.219433330000001 47.278354290000003 54.008953329999997 60.903713330000002 67.798473329999993 74.118669999999995;34.473799999999997 41.368560000000002 48.26332 55.158079999999998 62.052840000000003 68.947599999999994 75.842359999999999]  InternalRulePriority=Speed  RndMeth=Simplest
      settings: InputPortMap=u0,u1
  Constant : Constant  Value=car.prop_valve_pos
  p_rear_mod : Outport
  wires:
  P_rear/1 -> 2-D Lookup Table/1
  Constant/1 -> 2-D Lookup Table/2
  2-D Lookup Table/1 -> p_rear_mod/1

== system Vehicle_definitivo_validazione_2/Hardware in the Loop/Vehicle/Brakes/Rear Caliper ==
  P_rear : Inport
  Gain : Gain  Gain=2
  Pad Friction : Gain  Gain=car.brakepad_friction_coeff
  Piston area : Gain  Gain=car.area_rear_piston
  brake radius_rear : Gain  Gain=car.brake_radius_rear
  from bar to Pascal : Gain  Gain=100000
  T_brake_RR : Outport
  T_brake_RL : Outport  Port=2
  wires:
  P_rear/1 -> from bar to Pascal/1
  Pad Friction/1 -> brake radius_rear/1
  brake radius_rear/1 -> T_brake_RL/1, T_brake_RR/1
  from bar to Pascal/1 -> Gain/1
  Gain/1 -> Piston area/1
  Piston area/1 -> Pad Friction/1

== system Vehicle_definitivo_validazione_2/Hardware in the Loop/Vehicle/Chassis/Aeromaps ==
  Ride_height : Inport
  Constant : Constant  Value=car.Cx
  Constant1 : Constant  Value=car.Cz
  Constant2 : Constant  Value=car.x_cp
  Demux : Demux
  Mux : Mux  Inputs=3
  aero_coeff : Outport
  wires:
  Constant/1 -> Mux/1
  Constant1/1 -> Mux/2
  Ride_height/1 -> Demux/1
  Mux/1 -> aero_coeff/1
  Constant2/1 -> Mux/3

== system Vehicle_definitivo_validazione_2/Hardware in the Loop/Vehicle/Chassis/Damper ==
  susp_vel_ground : Inport
  IR : Inport  Port=2
  Demux : Demux
  FL : Subsystem
  FR : Subsystem
  Mux : Mux
  Product : Product
  Product1 : Product
  RL : Subsystem
  RR : Subsystem
  F_damper : Outport
  wires:
  IR/1 -> Product1/2, Product/2
  Product/1 -> Demux/1
  Demux/1 -> FR/1(V_FR)
  FR/1(F_FR) -> Mux/1  "F_FR"
  Mux/1 -> Product1/1
  Demux/2 -> FL/1(V_FL)
  FL/1(F_FL) -> Mux/2  "F_FL"
  Demux/3 -> RR/1(V_RR)
  RR/1(F_RR) -> Mux/3  "F_RR"
  Demux/4 -> RL/1(V_RL)
  RL/1(F_RL) -> Mux/4  "F_RL"
  susp_vel_ground/1 -> Product/1
  Product1/1 -> F_damper/1

== system Vehicle_definitivo_validazione_2/Hardware in the Loop/Vehicle/Chassis/kinematics ==
  Steer_Angle : Inport
  Wheel_Travel : Inport  Port=2
  Add{,1..5} (6 alike) : Sum
  Constant : Constant  Value=car.lf
  Constant1 : Constant  Value=car.lr
  Constant2 : Constant  Value=car.h_cog
  Constant3 : Constant  Value=0.03
  Constant4 : Constant  Value=0.04
  Degrees to Radians : simulink_extras/Transformations/Degrees to Radians
  Demux : Demux
  FL : Subsystem
  FR : Subsystem
  Gain{,1..3} (4 alike) : Gain  Gain=0.5
  Gain4 : Gain  Gain=-1
  Mux : Mux  Inputs=11
  Mux1 : Mux
  Mux2 : Mux
  Mux3 : Mux
  RL : Subsystem
  RR : Subsystem
  Subsystem : Subsystem
  Subsystem1 : Subsystem
  Subtract : Sum  Inputs=-+
  Subtract1 : Sum  Inputs=-+
  kin_dyn : Outport
  anti% : Outport  Port=2
  camber : Outport  Port=3
  toe : Outport  Port=4
  wires:
  Demux/1 -> FR/1(Wheel_Travel), Subtract/1, Add/1
  Add/1 -> Gain/1
  Gain/1 -> Subsystem/1(Heave_F)
  Subtract/1 -> Subsystem/2(Roll_F)
  Demux/3 -> Subtract1/1, Add1/1, RR/1(Wheel_Travel)
  Demux/4 -> RL/1(Wheel_Travel), Add1/2, Subtract1/2
  Add1/1 -> Gain1/1
  Steer_Angle/1 -> FR/2(Steer_Angle), Gain4/1
  Demux/2 -> FL/2(Wheel_Travel), Add/2, Subtract/2
  Mux/1 -> kin_dyn/1
  FR/3(IR_FR) -> Mux/1
  FL/3(IR_FL) -> Mux/2
  RR/3(IR_RR) -> Mux/3
  RL/3(IR_RL) -> Mux/4
  Subsystem/2(tf) -> Mux/5
  Subsystem1/2(tr) -> Mux/6
  FR/1(wb_FR) -> Add2/1
  FL/1(wb_FL) -> Add2/2
  Add2/1 -> Gain2/1
  Gain2/1 -> Add3/1
  Constant/1 -> Add3/2
  Add3/1 -> Mux/7
  Constant1/1 -> Add5/2
  Gain3/1 -> Add5/1
  Add4/1 -> Gain3/1
  Add5/1 -> Mux/8
  RR/1(wb_RR) -> Add4/1
  RL/1(wb_RL) -> Add4/2
  Constant2/1 -> Mux/9
  Mux3/1 -> Degrees to Radians/1
  Mux2/1 -> camber/1
  Mux1/1 -> anti%/1
  FR/2(AD_FR) -> Mux1/1
  FL/2(AD_FL) -> Mux1/2
  RR/2(AS_RR) -> Mux1/3
  RL/2(AS_RL) -> Mux1/4
  FR/4(Camber_FR) -> Mux2/1
  FL/4(Camber_FL) -> Mux2/2
  RR/4(Camber_RR) -> Mux2/3
  RL/4(Camber_RL) -> Mux2/4
  FR/5(Toe_FR) -> Mux3/1
  FL/5(Toe_FL) -> Mux3/2
  RR/5(Toe_RR) -> Mux3/3
  RL/5(Toe_RL) -> Mux3/4
  Gain4/1 -> FL/1(Steer_Angle)
  Constant3/1 -> Mux/10
  Constant4/1 -> Mux/11
  Subtract1/1 -> Subsystem1/2(Roll_R)
  Gain1/1 -> Subsystem1/1(Heave_R)
  Degrees to Radians/1 -> toe/1
  Wheel_Travel/1 -> Demux/1
